simulink model "Simulation_v2"  (R2020a)
settings: Solver=VariableStepAuto  StartTime=0.0  StopTime=tmax  RelTol=1e-3
values from neighbouring files (symbols this model uses):
  BPden = [1 alpha]    [RunSimulation.m]    (also in RunTest.m)
  BPnum = [0.3 alpha]    [RunSimulation.m]    (also in RunTest.m)
  c = 250    [RunSimulation.m]    (also in RunTest.m)
  fc = 0.45    [RunTest.m]
  Ft = 360000    [RunTest.m]
  l = 18    [RunSimulation.m]    (also in RunTest.m)
  num_wagons = 10    [RunTest.m]
  p0 = 0    [RunSimulation.m]    (also in RunTest.m)
  pool = readmatrix('pool.csv')    [RunTest.m]
  Pres = 0/1000*[5.7/771 0 1.6]    [RunSimulation.m]    (also in RunTest.m)
  RBD = 5    [RunSimulation.m]    (also in RunTest.m)
  tl = .1    (= 0.1)    [RunSimulation.m]    (also in RunTest.m)
  trackgradient = 0    [RunTest.m]
  v0 = 100/3.6    (= 27.7777777778)    [RunSimulation.m]
  VBD = 3.5    [RunSimulation.m]    (also in RunTest.m)
libraries: simulink x43, commrandsrc3 x40
(part 1 of 4)
settings Model: SimulationMode=accelerator  Creator=raphael  LastModifiedBy=Westfechtel
settings SolverCC: ZeroCrossControl=DisableAll
settings DataIOCC: ReturnWorkspaceOutputs=off
settings DebuggingCC: ArithmeticOperatorsInVariantConditions=warning
settings SFSimCC: CustomCodeUndefinedFunction=UseInterfaceOnly

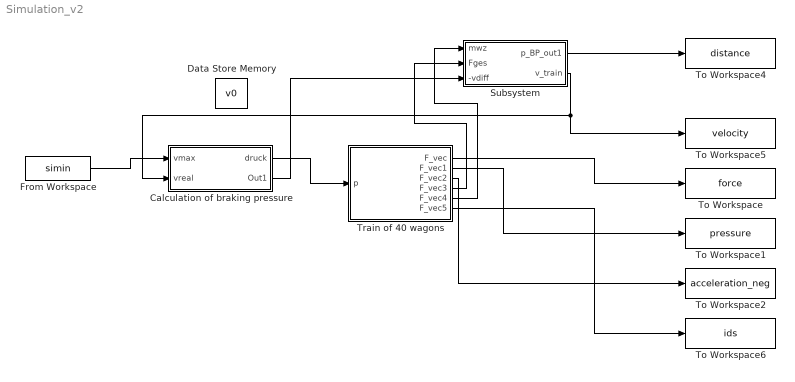
== system Simulation_v2 ==
  Calculation of braking pressure : Subsystem
  Data Store Memory : DataStoreMemory  DataStoreName=v0  ReadBeforeWriteMsg=warning  WriteAfterWriteMsg=warning  WriteAfterReadMsg=warning  ShowAdditionalParam=off
  From Workspace : FromWorkspace  VariableName=simin
  Subsystem : Subsystem
  To Workspace : ToWorkspace  VariableName=force  SaveFormat=Timeseries  SampleTime=-1
  To Workspace1 : ToWorkspace  VariableName=pressure  SaveFormat=Timeseries  SampleTime=-1
  To Workspace2 : ToWorkspace  VariableName=acceleration_neg  SaveFormat=Timeseries  SampleTime=-1
  To Workspace4 : ToWorkspace  VariableName=distance  SaveFormat=Timeseries  SampleTime=-1
  To Workspace5 : ToWorkspace  VariableName=velocity  SaveFormat=Timeseries  SampleTime=-1
  To Workspace6 : ToWorkspace  VariableName=ids  SampleTime=-1
  Train of 40 wagons : Subsystem
  wires:
  From Workspace/1 -> Calculation of braking pressure/1("vmax ")
  Calculation of braking pressure/1(druck) -> Train of 40 wagons/1(p)
  Subsystem/1(p_BP_out1) -> To Workspace4/1
  Subsystem/2(v_train) -> Calculation of braking pressure/2(vreal), To Workspace5/1
  Train of 40 wagons/1(F_vec) -> To Workspace/1
  Train of 40 wagons/2(F_vec1) -> To Workspace1/1
  Train of 40 wagons/3(F_vec2) -> To Workspace2/1
  Train of 40 wagons/4(F_vec3) -> Subsystem/2(Fges)
  Train of 40 wagons/5(F_vec4) -> Subsystem/1(mwz)
  Calculation of braking pressure/2(Out1) -> Subsystem/3("-vdiff ")
  Train of 40 wagons/6(F_vec5) -> To Workspace6/1

== system Simulation_v2/Calculation of braking pressure ==
  "vmax " : Inport
  vreal : Inport  Port=2
  1-D Lookup Table : Lookup_n-D  NumberOfTableDimensions=1  BreakpointsForDimension1=[1,2,5,10,15,20,25,30]  Table=[0.1,0.2,0.5,0.7,0.8,1,1.2,1.5]  InternalRulePriority=Speed  RndMeth=Simplest  InputSameDT=on
  Add : Sum  Inputs=+-
  Add1 : Sum
  Bias : Bias  Bias=-RBD
  Constant : Constant  Value=RBD
  Data Store Read : DataStoreRead  DataStoreName=v0
  Data Store Write : DataStoreWrite  DataStoreName=v0
  Detect Decrease : simulink/Logic and Bit Operations/Detect Decrease  vinit=0.0  OutDataTypeStr=boolean
  Divide : Product  Inputs=**
  Divide1 : Product  Inputs=**
  Gain : Gain  Gain=-1
  Logical Operator : Logic  Operator=NOT  Inputs=1  AllPortsSameDT=off  OutDataTypeStr=boolean
  Product : Product
  Relational Operator : RelationalOperator  Operator=>  OutDataTypeStr=boolean  RndMeth=Simplest
  Subtract : Sum  Inputs=+-
  To Workspace : ToWorkspace  VariableName=v0_out  SaveFormat=Timeseries  SampleTime=-1
  druck : Outport
  Out1 : Outport  Port=2
  wires:
  "vmax "/1 -> Subtract/2, Detect Decrease/1, Relational Operator/2
  Constant/1 -> Add/1
  Add/1 -> Bias/1
  Bias/1 -> druck/1
  Detect Decrease/1 -> Logical Operator/1, Divide/2
  Logical Operator/1 -> Divide1/1
  Data Store Read/1 -> Divide1/2
  Divide/1 -> Add1/1
  Divide1/1 -> Add1/2
  Add1/1 -> To Workspace/1, Data Store Write/1
  vreal/1 -> Relational Operator/1, Subtract/1, Divide/1
  Relational Operator/1 -> Product/1
  Subtract/1 -> Gain/1, 1-D Lookup Table/1
  1-D Lookup Table/1 -> Product/2
  Product/1 -> Add/2
  Gain/1 -> Out1/1

== system Simulation_v2/Subsystem ==
  mwz : Inport
  Fges : Inport  Port=2
  "-vdiff " : Inport  Port=3
  1-D Lookup Table : Lookup_n-D  NumberOfTableDimensions=1  BreakpointsForDimension1=[1,2,5,10,15,20,25,30]  Table=[0.05,0.1,0.15,0.3,0.45,0.6,0.85,1]  InternalRulePriority=Speed  RndMeth=Simplest  InputSameDT=on
  Add : Sum
  Compare To Zero : simulink/Logic and Bit Operations/Compare To Zero  relop=~=  OutDataTypeStr=boolean
  Compare To Zero1 : simulink/Logic and Bit Operations/Compare To Zero  relop===  OutDataTypeStr=boolean
  Constant : Constant  Value=Ft
  Data Store Read : DataStoreRead  DataStoreName=v0
  Dead Zone : DeadZone  LowerValue=-0.05  UpperValue=0.05  SaturateOnIntegerOverflow=on
  Divide1 : Product  Inputs=**
  Divide2 : Product  Inputs=**
  Divide3 : Product  Inputs=**
  Integrator : Integrator  InitialConditionSource=external  InitialCondition=v0
  Integrator1 : Integrator
  Mux4 : Mux  Inputs=1
  a=F/m : Product  Inputs=*/
  p_BP_out1 : Outport  VectorParamsAs1DForOutWhenUnconnected=off
  v_train : Outport  Port=2
  wires:
  Integrator1/1 -> Mux4/1
  Integrator/1 -> v_train/1, Integrator1/1  "v"
  a=F/m/1 -> Integrator/1  "a"
  Mux4/1 -> p_BP_out1/1  "distance_vec"
  mwz/1 -> a=F/m/2
  Data Store Read/1 -> Integrator/2
  Fges/1 -> Dead Zone/1
  Compare To Zero/1 -> Divide1/1
  Compare To Zero1/1 -> Divide2/2
  Divide1/1 -> Add/2
  Add/1 -> a=F/m/1
  Dead Zone/1 -> Compare To Zero1/1, Compare To Zero/1, Divide1/2
  Divide2/1 -> Add/1
  "-vdiff "/1 -> 1-D Lookup Table/1
  1-D Lookup Table/1 -> Divide3/2
  Divide3/1 -> Divide2/1
  Constant/1 -> Divide3/1

== system Simulation_v2/Train of 40 wagons ==
  p : Inport
  Add : Sum  Inputs=++++++++
  Add1 : Sum  Inputs=++++++++
  Mux{,1..3} (4 alike) : Mux  Inputs=8
  Subsystem1 : Subsystem
  Subsystem2 : Subsystem
  Subsystem3 : Subsystem
  Subsystem4 : Subsystem
  Subsystem5 : Subsystem
  Subsystem6 : Subsystem
  Subsystem7 : Subsystem
  Subsystem8 : Subsystem
  Terminator : Terminator
  F_vec : Outport  VectorParamsAs1DForOutWhenUnconnected=off
  F_vec1 : Outport  Port=2  VectorParamsAs1DForOutWhenUnconnected=off
  F_vec2 : Outport  Port=3  VectorParamsAs1DForOutWhenUnconnected=off
  F_vec3 : Outport  Port=4  VectorParamsAs1DForOutWhenUnconnected=off
  F_vec4 : Outport  Port=5  VectorParamsAs1DForOutWhenUnconnected=off
  F_vec5 : Outport  Port=6  VectorParamsAs1DForOutWhenUnconnected=off
  wires:
  p/1 -> Subsystem1/1(In1)
  Mux/1 -> F_vec/1  "F_vec"
  Mux1/1 -> F_vec1/1  "BP_vec"
  Mux2/1 -> F_vec2/1  "ares_vec"
  Add/1 -> F_vec3/1  "Fges"
  Add1/1 -> F_vec4/1  "mwz"
  Subsystem1/1(F_vec) -> Mux/1
  Subsystem2/1(F_vec) -> Mux/2
  Subsystem3/1(F_vec) -> Mux/3
  Subsystem4/1(F_vec) -> Mux/4
  Subsystem5/1(F_vec) -> Mux/5
  Subsystem6/1(F_vec) -> Mux/6
  Subsystem8/1(F_vec) -> Mux/7
  Subsystem7/1(F_vec) -> Mux/8
  Subsystem1/2(BP_vec) -> Mux1/1
  Subsystem2/2(BP_vec) -> Mux1/2
  Subsystem3/2(BP_vec) -> Mux1/3
  Subsystem4/2(BP_vec) -> Mux1/4
  Subsystem5/2(BP_vec) -> Mux1/5
  Subsystem6/2(BP_vec) -> Mux1/6
  Subsystem8/2(BP_vec) -> Mux1/7
  Subsystem7/2(BP_vec) -> Mux1/8
  Subsystem1/3(ares_vec) -> Mux2/1
  Subsystem2/3(ares_vec) -> Mux2/2
  Subsystem3/3(ares_vec) -> Mux2/3
  Subsystem4/3(ares_vec) -> Mux2/4
  Subsystem5/3(ares_vec) -> Mux2/5
  Subsystem6/3(ares_vec) -> Mux2/6
  Subsystem8/3(ares_vec) -> Mux2/7
  Subsystem7/3(ares_vec) -> Mux2/8
  Subsystem1/4(p_BP_out) -> Subsystem2/1(In1)
  Subsystem2/4(p_BP_out) -> Subsystem3/1(In1)
  Subsystem3/4(p_BP_out) -> Subsystem4/1(In1)
  Subsystem4/4(p_BP_out) -> Subsystem5/1(In1)
  Subsystem5/4(p_BP_out) -> Subsystem6/1(In1)
  Subsystem6/4(p_BP_out) -> Subsystem8/1(In1)
  Subsystem8/4(p_BP_out) -> Subsystem7/1(In1)
  Subsystem7/4(p_BP_out) -> Terminator/1
  Subsystem1/5(BP_vec1) -> Add/1
  Subsystem2/5(BP_vec1) -> Add/2
  Subsystem3/5(BP_vec1) -> Add/3
  Subsystem4/5(BP_vec1) -> Add/4
  Subsystem5/5(BP_vec1) -> Add/5
  Subsystem6/5(BP_vec1) -> Add/6
  Subsystem8/5(BP_vec1) -> Add/7
  Subsystem7/5(BP_vec1) -> Add/8
  Subsystem1/6(BP_vec2) -> Add1/1
  Subsystem2/6(BP_vec2) -> Add1/2
  Subsystem3/6(BP_vec2) -> Add1/3
  Subsystem4/6(BP_vec2) -> Add1/4
  Subsystem5/6(BP_vec2) -> Add1/5
  Subsystem6/6(BP_vec2) -> Add1/6
  Subsystem8/6(BP_vec2) -> Add1/7
  Subsystem7/6(BP_vec2) -> Add1/8
  Mux3/1 -> F_vec5/1  "id_vec"
  Subsystem1/7(ares_vec1) -> Mux3/1
  Subsystem2/7(ares_vec1) -> Mux3/2
  Subsystem3/7(ares_vec1) -> Mux3/3
  Subsystem4/7(ares_vec1) -> Mux3/4
  Subsystem5/7(ares_vec1) -> Mux3/5
  Subsystem6/7(ares_vec1) -> Mux3/6
  Subsystem8/7(ares_vec1) -> Mux3/7
  Subsystem7/7(ares_vec1) -> Mux3/8

== system Simulation_v2/Train of 40 wagons/Subsystem1 ==
  In1 : Inport
  Add : Sum  Inputs=+++++
  Add1 : Sum  Inputs=+++++
  Mux{,1..3} (4 alike) : Mux  Inputs=5
  Wagon model1 : Subsystem
  Wagon model2 : Subsystem
  Wagon model3 : Subsystem
  Wagon model4 : Subsystem
  Wagon model5 : Subsystem
  F_vec : Outport  VectorParamsAs1DForOutWhenUnconnected=off
  BP_vec : Outport  Port=2  VectorParamsAs1DForOutWhenUnconnected=off
  ares_vec : Outport  Port=3  VectorParamsAs1DForOutWhenUnconnected=off
  p_BP_out : Outport  Port=4  VectorParamsAs1DForOutWhenUnconnected=off
  BP_vec1 : Outport  Port=5  VectorParamsAs1DForOutWhenUnconnected=off
  BP_vec2 : Outport  Port=6  VectorParamsAs1DForOutWhenUnconnected=off
  ares_vec1 : Outport  Port=7  VectorParamsAs1DForOutWhenUnconnected=off
  wires:
  In1/1 -> Wagon model5/1(p)
  Mux1/1 -> BP_vec/1  "BP_vec"
  Mux/1 -> F_vec/1  "F_vec"
  Mux3/1 -> ares_vec/1  "ares_vec"
  Add1/1 -> BP_vec2/1  "msum"
  Add/1 -> BP_vec1/1  "Fsum"
  Wagon model5/2(p_BP_out) -> Wagon model3/1(p), Mux1/1  "p_BP_out"
  Wagon model3/2(p_BP_out) -> Wagon model2/1(p), Mux1/2  "p_BP_out"
  Wagon model2/2(p_BP_out) -> Wagon model1/1(p), Mux1/3  "p_BP_out"
  Wagon model1/2(p_BP_out) -> Wagon model4/1(p), Mux1/4  "p_BP_out"
  Wagon model4/2(p_BP_out) -> Mux1/5, p_BP_out/1  "p_BP_out"
  Wagon model5/1(Fres) -> Add/1, Mux/1
  Wagon model3/1(Fres) -> Add/2, Mux/2
  Wagon model2/1(Fres) -> Mux/3, Add/3
  Wagon model1/1(Fres) -> Mux/4, Add/4
  Wagon model4/1(Fres) -> Mux/5, Add/5
  Wagon model5/3(ares) -> Mux3/1
  Wagon model3/3(ares) -> Mux3/2
  Wagon model2/3(ares) -> Mux3/3
  Wagon model1/3(ares) -> Mux3/4
  Wagon model4/3(ares) -> Mux3/5
  Wagon model5/4(m) -> Add1/1
  Wagon model3/4(m) -> Add1/2
  Wagon model2/4(m) -> Add1/3
  Wagon model1/4(m) -> Add1/4
  Wagon model4/4(m) -> Add1/5
  Mux2/1 -> ares_vec1/1  "id_vec"
  Wagon model5/5("id ") -> Mux2/1
  Wagon model3/5("id ") -> Mux2/2
  Wagon model2/5("id ") -> Mux2/3
  Wagon model1/5("id ") -> Mux2/4
  Wagon model4/5("id ") -> Mux2/5

== system Simulation_v2/Train of 40 wagons/Subsystem2 ==
  In1 : Inport
  Add : Sum  Inputs=+++++
  Add1 : Sum  Inputs=+++++
  Mux{,1..3} (4 alike) : Mux  Inputs=5
  Wagon model1 : Subsystem
  Wagon model2 : Subsystem
  Wagon model3 : Subsystem
  Wagon model4 : Subsystem
  Wagon model5 : Subsystem
  F_vec : Outport  VectorParamsAs1DForOutWhenUnconnected=off
  BP_vec : Outport  Port=2  VectorParamsAs1DForOutWhenUnconnected=off
  ares_vec : Outport  Port=3  VectorParamsAs1DForOutWhenUnconnected=off
  p_BP_out : Outport  Port=4  VectorParamsAs1DForOutWhenUnconnected=off
  BP_vec1 : Outport  Port=5  VectorParamsAs1DForOutWhenUnconnected=off
  BP_vec2 : Outport  Port=6  VectorParamsAs1DForOutWhenUnconnected=off
  ares_vec1 : Outport  Port=7  VectorParamsAs1DForOutWhenUnconnected=off
  wires:
  In1/1 -> Wagon model5/1(p)
  Mux1/1 -> BP_vec/1  "BP_vec"
  Mux/1 -> F_vec/1  "F_vec"
  Mux3/1 -> ares_vec/1  "ares_vec"
  Add1/1 -> BP_vec2/1  "msum"
  Add/1 -> BP_vec1/1  "Fsum"
  Wagon model5/2(p_BP_out) -> Wagon model3/1(p), Mux1/1  "p_BP_out"
  Wagon model3/2(p_BP_out) -> Wagon model2/1(p), Mux1/2  "p_BP_out"
  Wagon model2/2(p_BP_out) -> Wagon model1/1(p), Mux1/3  "p_BP_out"
  Wagon model1/2(p_BP_out) -> Wagon model4/1(p), Mux1/4  "p_BP_out"
  Wagon model4/2(p_BP_out) -> Mux1/5, p_BP_out/1  "p_BP_out"
  Wagon model5/1(Fres) -> Add/1, Mux/1
  Wagon model3/1(Fres) -> Add/2, Mux/2
  Wagon model2/1(Fres) -> Mux/3, Add/3
  Wagon model1/1(Fres) -> Mux/4, Add/4
  Wagon model4/1(Fres) -> Mux/5, Add/5
  Wagon model5/3(ares) -> Mux3/1
  Wagon model3/3(ares) -> Mux3/2
  Wagon model2/3(ares) -> Mux3/3
  Wagon model1/3(ares) -> Mux3/4
  Wagon model4/3(ares) -> Mux3/5
  Wagon model5/4(m) -> Add1/1
  Wagon model3/4(m) -> Add1/2
  Wagon model2/4(m) -> Add1/3
  Wagon model1/4(m) -> Add1/4
  Wagon model4/4(m) -> Add1/5
  Mux2/1 -> ares_vec1/1  "id_vec"
  Wagon model5/5("id ") -> Mux2/1
  Wagon model3/5("id ") -> Mux2/2
  Wagon model2/5("id ") -> Mux2/3
  Wagon model1/5("id ") -> Mux2/4
  Wagon model4/5("id ") -> Mux2/5

== system Simulation_v2/Train of 40 wagons/Subsystem3 ==
  In1 : Inport
  Add : Sum  Inputs=+++++
  Add1 : Sum  Inputs=+++++
  Mux{,1..3} (4 alike) : Mux  Inputs=5
  Wagon model1 : Subsystem
  Wagon model2 : Subsystem
  Wagon model3 : Subsystem
  Wagon model4 : Subsystem
  Wagon model5 : Subsystem
  F_vec : Outport  VectorParamsAs1DForOutWhenUnconnected=off
  BP_vec : Outport  Port=2  VectorParamsAs1DForOutWhenUnconnected=off
  ares_vec : Outport  Port=3  VectorParamsAs1DForOutWhenUnconnected=off
  p_BP_out : Outport  Port=4  VectorParamsAs1DForOutWhenUnconnected=off
  BP_vec1 : Outport  Port=5  VectorParamsAs1DForOutWhenUnconnected=off
  BP_vec2 : Outport  Port=6  VectorParamsAs1DForOutWhenUnconnected=off
  ares_vec1 : Outport  Port=7  VectorParamsAs1DForOutWhenUnconnected=off
  wires:
  In1/1 -> Wagon model5/1(p)
  Mux1/1 -> BP_vec/1  "BP_vec"
  Mux/1 -> F_vec/1  "F_vec"
  Mux3/1 -> ares_vec/1  "ares_vec"
  Add1/1 -> BP_vec2/1  "msum"
  Add/1 -> BP_vec1/1  "Fsum"
  Wagon model5/2(p_BP_out) -> Wagon model3/1(p), Mux1/1  "p_BP_out"
  Wagon model3/2(p_BP_out) -> Wagon model2/1(p), Mux1/2  "p_BP_out"
  Wagon model2/2(p_BP_out) -> Wagon model1/1(p), Mux1/3  "p_BP_out"
  Wagon model1/2(p_BP_out) -> Wagon model4/1(p), Mux1/4  "p_BP_out"
  Wagon model4/2(p_BP_out) -> Mux1/5, p_BP_out/1  "p_BP_out"
  Wagon model5/1(Fres) -> Add/1, Mux/1
  Wagon model3/1(Fres) -> Add/2, Mux/2
  Wagon model2/1(Fres) -> Mux/3, Add/3
  Wagon model1/1(Fres) -> Mux/4, Add/4
  Wagon model4/1(Fres) -> Mux/5, Add/5
  Wagon model5/3(ares) -> Mux3/1
  Wagon model3/3(ares) -> Mux3/2
  Wagon model2/3(ares) -> Mux3/3
  Wagon model1/3(ares) -> Mux3/4
  Wagon model4/3(ares) -> Mux3/5
  Wagon model5/4(m) -> Add1/1
  Wagon model3/4(m) -> Add1/2
  Wagon model2/4(m) -> Add1/3
  Wagon model1/4(m) -> Add1/4
  Wagon model4/4(m) -> Add1/5
  Mux2/1 -> ares_vec1/1  "id_vec"
  Wagon model5/5("id ") -> Mux2/1
  Wagon model3/5("id ") -> Mux2/2
  Wagon model2/5("id ") -> Mux2/3
  Wagon model1/5("id ") -> Mux2/4
  Wagon model4/5("id ") -> Mux2/5

== system Simulation_v2/Train of 40 wagons/Subsystem4 ==
  In1 : Inport
  Add : Sum  Inputs=+++++
  Add1 : Sum  Inputs=+++++
  Mux{,1..3} (4 alike) : Mux  Inputs=5
  Wagon model1 : Subsystem
  Wagon model2 : Subsystem
  Wagon model3 : Subsystem
  Wagon model4 : Subsystem
  Wagon model5 : Subsystem
  F_vec : Outport  VectorParamsAs1DForOutWhenUnconnected=off
  BP_vec : Outport  Port=2  VectorParamsAs1DForOutWhenUnconnected=off
  ares_vec : Outport  Port=3  VectorParamsAs1DForOutWhenUnconnected=off
  p_BP_out : Outport  Port=4  VectorParamsAs1DForOutWhenUnconnected=off
  BP_vec1 : Outport  Port=5  VectorParamsAs1DForOutWhenUnconnected=off
  BP_vec2 : Outport  Port=6  VectorParamsAs1DForOutWhenUnconnected=off
  ares_vec1 : Outport  Port=7  VectorParamsAs1DForOutWhenUnconnected=off
  wires:
  In1/1 -> Wagon model5/1(p)
  Mux1/1 -> BP_vec/1  "BP_vec"
  Mux/1 -> F_vec/1  "F_vec"
  Mux3/1 -> ares_vec/1  "ares_vec"
  Add1/1 -> BP_vec2/1  "msum"
  Add/1 -> BP_vec1/1  "Fsum"
  Wagon model5/2(p_BP_out) -> Wagon model3/1(p), Mux1/1  "p_BP_out"
  Wagon model3/2(p_BP_out) -> Wagon model2/1(p), Mux1/2  "p_BP_out"
  Wagon model2/2(p_BP_out) -> Wagon model1/1(p), Mux1/3  "p_BP_out"
  Wagon model1/2(p_BP_out) -> Wagon model4/1(p), Mux1/4  "p_BP_out"
  Wagon model4/2(p_BP_out) -> Mux1/5, p_BP_out/1  "p_BP_out"
  Wagon model5/1(Fres) -> Add/1, Mux/1
  Wagon model3/1(Fres) -> Add/2, Mux/2
  Wagon model2/1(Fres) -> Mux/3, Add/3
  Wagon model1/1(Fres) -> Mux/4, Add/4
  Wagon model4/1(Fres) -> Mux/5, Add/5
  Wagon model5/3(ares) -> Mux3/1
  Wagon model3/3(ares) -> Mux3/2
  Wagon model2/3(ares) -> Mux3/3
  Wagon model1/3(ares) -> Mux3/4
  Wagon model4/3(ares) -> Mux3/5
  Wagon model5/4(m) -> Add1/1
  Wagon model3/4(m) -> Add1/2
  Wagon model2/4(m) -> Add1/3
  Wagon model1/4(m) -> Add1/4
  Wagon model4/4(m) -> Add1/5
  Mux2/1 -> ares_vec1/1  "id_vec"
  Wagon model5/5("id ") -> Mux2/1
  Wagon model3/5("id ") -> Mux2/2
  Wagon model2/5("id ") -> Mux2/3
  Wagon model1/5("id ") -> Mux2/4
  Wagon model4/5("id ") -> Mux2/5

== system Simulation_v2/Train of 40 wagons/Subsystem5 ==
  In1 : Inport
  Add : Sum  Inputs=+++++
  Add1 : Sum  Inputs=+++++
  Mux{,1..3} (4 alike) : Mux  Inputs=5
  Wagon model1 : Subsystem
  Wagon model2 : Subsystem
  Wagon model3 : Subsystem
  Wagon model4 : Subsystem
  Wagon model5 : Subsystem
  F_vec : Outport  VectorParamsAs1DForOutWhenUnconnected=off
  BP_vec : Outport  Port=2  VectorParamsAs1DForOutWhenUnconnected=off
  ares_vec : Outport  Port=3  VectorParamsAs1DForOutWhenUnconnected=off
  p_BP_out : Outport  Port=4  VectorParamsAs1DForOutWhenUnconnected=off
  BP_vec1 : Outport  Port=5  VectorParamsAs1DForOutWhenUnconnected=off
  BP_vec2 : Outport  Port=6  VectorParamsAs1DForOutWhenUnconnected=off
  ares_vec1 : Outport  Port=7  VectorParamsAs1DForOutWhenUnconnected=off
  wires:
  In1/1 -> Wagon model5/1(p)
  Mux1/1 -> BP_vec/1  "BP_vec"
  Mux/1 -> F_vec/1  "F_vec"
  Mux3/1 -> ares_vec/1  "ares_vec"
  Add1/1 -> BP_vec2/1  "msum"
  Add/1 -> BP_vec1/1  "Fsum"
  Wagon model5/2(p_BP_out) -> Wagon model3/1(p), Mux1/1  "p_BP_out"
  Wagon model3/2(p_BP_out) -> Wagon model2/1(p), Mux1/2  "p_BP_out"
  Wagon model2/2(p_BP_out) -> Wagon model1/1(p), Mux1/3  "p_BP_out"
  Wagon model1/2(p_BP_out) -> Wagon model4/1(p), Mux1/4  "p_BP_out"
  Wagon model4/2(p_BP_out) -> Mux1/5, p_BP_out/1  "p_BP_out"
  Wagon model5/1(Fres) -> Add/1, Mux/1
  Wagon model3/1(Fres) -> Add/2, Mux/2
  Wagon model2/1(Fres) -> Mux/3, Add/3
  Wagon model1/1(Fres) -> Mux/4, Add/4
  Wagon model4/1(Fres) -> Mux/5, Add/5
  Wagon model5/3(ares) -> Mux3/1
  Wagon model3/3(ares) -> Mux3/2
  Wagon model2/3(ares) -> Mux3/3
  Wagon model1/3(ares) -> Mux3/4
  Wagon model4/3(ares) -> Mux3/5
  Wagon model5/4(m) -> Add1/1
  Wagon model3/4(m) -> Add1/2
  Wagon model2/4(m) -> Add1/3
  Wagon model1/4(m) -> Add1/4
  Wagon model4/4(m) -> Add1/5
  Mux2/1 -> ares_vec1/1  "id_vec"
  Wagon model5/5("id ") -> Mux2/1
  Wagon model3/5("id ") -> Mux2/2
  Wagon model2/5("id ") -> Mux2/3
  Wagon model1/5("id ") -> Mux2/4
  Wagon model4/5("id ") -> Mux2/5

== system Simulation_v2/Train of 40 wagons/Subsystem6 ==
  In1 : Inport
  Add : Sum  Inputs=+++++
  Add1 : Sum  Inputs=+++++
  Mux{,1..3} (4 alike) : Mux  Inputs=5
  Wagon model1 : Subsystem
  Wagon model2 : Subsystem
  Wagon model3 : Subsystem
  Wagon model4 : Subsystem
  Wagon model5 : Subsystem
  F_vec : Outport  VectorParamsAs1DForOutWhenUnconnected=off
  BP_vec : Outport  Port=2  VectorParamsAs1DForOutWhenUnconnected=off
  ares_vec : Outport  Port=3  VectorParamsAs1DForOutWhenUnconnected=off
  p_BP_out : Outport  Port=4  VectorParamsAs1DForOutWhenUnconnected=off
  BP_vec1 : Outport  Port=5  VectorParamsAs1DForOutWhenUnconnected=off
  BP_vec2 : Outport  Port=6  VectorParamsAs1DForOutWhenUnconnected=off
  ares_vec1 : Outport  Port=7  VectorParamsAs1DForOutWhenUnconnected=off
  wires:
  In1/1 -> Wagon model5/1(p)
  Mux1/1 -> BP_vec/1  "BP_vec"
  Mux/1 -> F_vec/1  "F_vec"
  Mux3/1 -> ares_vec/1  "ares_vec"
  Add1/1 -> BP_vec2/1  "msum"
  Add/1 -> BP_vec1/1  "Fsum"
  Wagon model5/2(p_BP_out) -> Wagon model3/1(p), Mux1/1  "p_BP_out"
  Wagon model3/2(p_BP_out) -> Wagon model2/1(p), Mux1/2  "p_BP_out"
  Wagon model2/2(p_BP_out) -> Wagon model1/1(p), Mux1/3  "p_BP_out"
  Wagon model1/2(p_BP_out) -> Wagon model4/1(p), Mux1/4  "p_BP_out"
  Wagon model4/2(p_BP_out) -> Mux1/5, p_BP_out/1  "p_BP_out"
  Wagon model5/1(Fres) -> Add/1, Mux/1
  Wagon model3/1(Fres) -> Add/2, Mux/2
  Wagon model2/1(Fres) -> Mux/3, Add/3
  Wagon model1/1(Fres) -> Mux/4, Add/4
  Wagon model4/1(Fres) -> Mux/5, Add/5
  Wagon model5/3(ares) -> Mux3/1
  Wagon model3/3(ares) -> Mux3/2
  Wagon model2/3(ares) -> Mux3/3
  Wagon model1/3(ares) -> Mux3/4
  Wagon model4/3(ares) -> Mux3/5
  Wagon model5/4(m) -> Add1/1
  Wagon model3/4(m) -> Add1/2
  Wagon model2/4(m) -> Add1/3
  Wagon model1/4(m) -> Add1/4
  Wagon model4/4(m) -> Add1/5
  Mux2/1 -> ares_vec1/1  "id_vec"
  Wagon model5/5("id ") -> Mux2/1
  Wagon model3/5("id ") -> Mux2/2
  Wagon model2/5("id ") -> Mux2/3
  Wagon model1/5("id ") -> Mux2/4
  Wagon model4/5("id ") -> Mux2/5

== system Simulation_v2/Train of 40 wagons/Subsystem7 ==
  In1 : Inport
  Add : Sum  Inputs=+++++
  Add1 : Sum  Inputs=+++++
  Mux{,1..3} (4 alike) : Mux  Inputs=5
  Wagon model1 : Subsystem
  Wagon model2 : Subsystem
  Wagon model3 : Subsystem
  Wagon model4 : Subsystem
  Wagon model5 : Subsystem
  F_vec : Outport  VectorParamsAs1DForOutWhenUnconnected=off
  BP_vec : Outport  Port=2  VectorParamsAs1DForOutWhenUnconnected=off
  ares_vec : Outport  Port=3  VectorParamsAs1DForOutWhenUnconnected=off
  p_BP_out : Outport  Port=4  VectorParamsAs1DForOutWhenUnconnected=off
  BP_vec1 : Outport  Port=5  VectorParamsAs1DForOutWhenUnconnected=off
  BP_vec2 : Outport  Port=6  VectorParamsAs1DForOutWhenUnconnected=off
  ares_vec1 : Outport  Port=7  VectorParamsAs1DForOutWhenUnconnected=off
  wires:
  In1/1 -> Wagon model5/1(p)
  Mux1/1 -> BP_vec/1  "BP_vec"
  Mux/1 -> F_vec/1  "F_vec"
  Mux3/1 -> ares_vec/1  "ares_vec"
  Add1/1 -> BP_vec2/1  "msum"
  Add/1 -> BP_vec1/1  "Fsum"
  Wagon model5/2(p_BP_out) -> Wagon model3/1(p), Mux1/1  "p_BP_out"
  Wagon model3/2(p_BP_out) -> Wagon model2/1(p), Mux1/2  "p_BP_out"
  Wagon model2/2(p_BP_out) -> Wagon model1/1(p), Mux1/3  "p_BP_out"
  Wagon model1/2(p_BP_out) -> Wagon model4/1(p), Mux1/4  "p_BP_out"
  Wagon model4/2(p_BP_out) -> Mux1/5, p_BP_out/1  "p_BP_out"
  Wagon model5/1(Fres) -> Add/1, Mux/1
  Wagon model3/1(Fres) -> Add/2, Mux/2
  Wagon model2/1(Fres) -> Mux/3, Add/3
  Wagon model1/1(Fres) -> Mux/4, Add/4
  Wagon model4/1(Fres) -> Mux/5, Add/5
  Wagon model5/3(ares) -> Mux3/1
  Wagon model3/3(ares) -> Mux3/2
  Wagon model2/3(ares) -> Mux3/3
  Wagon model1/3(ares) -> Mux3/4
  Wagon model4/3(ares) -> Mux3/5
  Wagon model5/4(m) -> Add1/1
  Wagon model3/4(m) -> Add1/2
  Wagon model2/4(m) -> Add1/3
  Wagon model1/4(m) -> Add1/4
  Wagon model4/4(m) -> Add1/5
  Mux2/1 -> ares_vec1/1  "id_vec"
  Wagon model5/5("id ") -> Mux2/1
  Wagon model3/5("id ") -> Mux2/2
  Wagon model2/5("id ") -> Mux2/3
  Wagon model1/5("id ") -> Mux2/4
  Wagon model4/5("id ") -> Mux2/5

== system Simulation_v2/Train of 40 wagons/Subsystem8 ==
  In1 : Inport
  Add : Sum  Inputs=+++++
  Add1 : Sum  Inputs=+++++
  Mux{,1..3} (4 alike) : Mux  Inputs=5
  Wagon model1 : Subsystem
  Wagon model2 : Subsystem
  Wagon model3 : Subsystem
  Wagon model4 : Subsystem
  Wagon model5 : Subsystem
  F_vec : Outport  VectorParamsAs1DForOutWhenUnconnected=off
  BP_vec : Outport  Port=2  VectorParamsAs1DForOutWhenUnconnected=off
  ares_vec : Outport  Port=3  VectorParamsAs1DForOutWhenUnconnected=off
  p_BP_out : Outport  Port=4  VectorParamsAs1DForOutWhenUnconnected=off
  BP_vec1 : Outport  Port=5  VectorParamsAs1DForOutWhenUnconnected=off
  BP_vec2 : Outport  Port=6  VectorParamsAs1DForOutWhenUnconnected=off
  ares_vec1 : Outport  Port=7  VectorParamsAs1DForOutWhenUnconnected=off
  wires:
  In1/1 -> Wagon model5/1(p)
  Mux1/1 -> BP_vec/1  "BP_vec"
  Mux/1 -> F_vec/1  "F_vec"
  Mux3/1 -> ares_vec/1  "ares_vec"
  Add1/1 -> BP_vec2/1  "msum"
  Add/1 -> BP_vec1/1  "Fsum"
  Wagon model5/2(p_BP_out) -> Wagon model3/1(p), Mux1/1  "p_BP_out"
  Wagon model3/2(p_BP_out) -> Wagon model2/1(p), Mux1/2  "p_BP_out"
  Wagon model2/2(p_BP_out) -> Wagon model1/1(p), Mux1/3  "p_BP_out"
  Wagon model1/2(p_BP_out) -> Wagon model4/1(p), Mux1/4  "p_BP_out"
  Wagon model4/2(p_BP_out) -> Mux1/5, p_BP_out/1  "p_BP_out"
  Wagon model5/1(Fres) -> Add/1, Mux/1
  Wagon model3/1(Fres) -> Add/2, Mux/2
  Wagon model2/1(Fres) -> Mux/3, Add/3
  Wagon model1/1(Fres) -> Mux/4, Add/4
  Wagon model4/1(Fres) -> Mux/5, Add/5
  Wagon model5/3(ares) -> Mux3/1
  Wagon model3/3(ares) -> Mux3/2
  Wagon model2/3(ares) -> Mux3/3
  Wagon model1/3(ares) -> Mux3/4
  Wagon model4/3(ares) -> Mux3/5
  Wagon model5/4(m) -> Add1/1
  Wagon model3/4(m) -> Add1/2
  Wagon model2/4(m) -> Add1/3
  Wagon model1/4(m) -> Add1/4
  Wagon model4/4(m) -> Add1/5
  Mux2/1 -> ares_vec1/1  "id_vec"
  Wagon model5/5("id ") -> Mux2/1
  Wagon model3/5("id ") -> Mux2/2
  Wagon model2/5("id ") -> Mux2/3
  Wagon model1/5("id ") -> Mux2/4
  Wagon model4/5("id ") -> Mux2/5

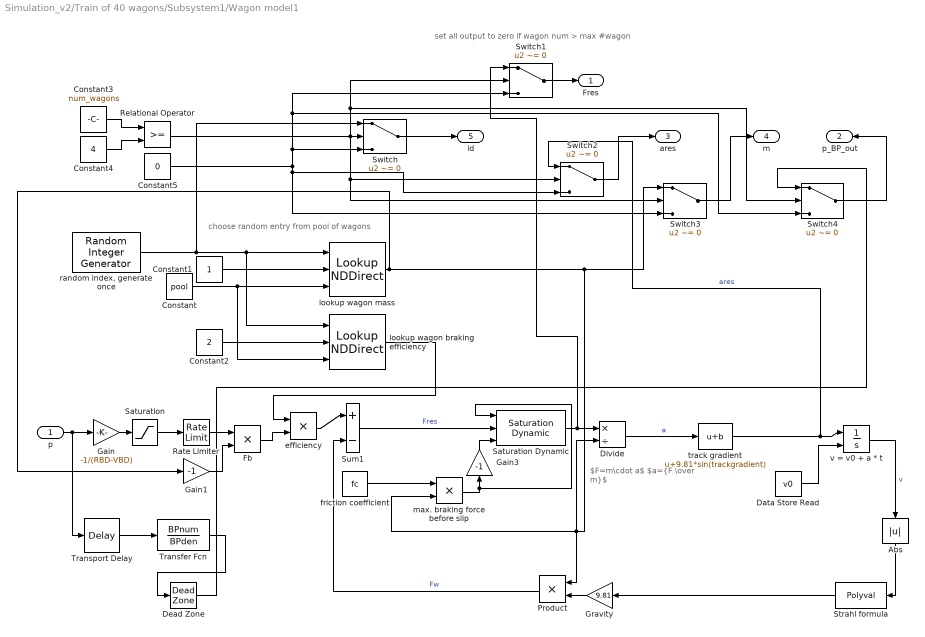
== system Simulation_v2/Train of 40 wagons/Subsystem1/Wagon model1 ==
  note: set all output to zero if wagon num > max #wagon
  note: choose random entry from pool of wagons
  note: $F=m\cdot a$ $a={F \over m}$
  p : Inport
  Abs : Abs
  Constant : Constant  Value=pool
  Constant1 : Constant
  Constant2 : Constant  Value=2
  Constant3 : Constant  Value=num_wagons
  Constant4 : Constant  Value=4
  Constant5 : Constant  Value=0  OutDataTypeStr=uint32
  Data Store Read : DataStoreRead  DataStoreName=v0
  Dead Zone : DeadZone  LowerValue=-0.005  UpperValue=0.005  SaturateOnIntegerOverflow=on
  Divide : Product  Inputs=*/
  Fb : Product  Inputs=**
  Gain : Gain  Gain=-1/(RBD-VBD)
  Gain1 : Gain  Gain=-1
  Gain3 : Gain  Gain=-1
  Gravity : Gain  Gain=9.81
  Product : Product
  Rate Limiter : RateLimiter  RisingSlewLimit=1/tf  FallingSlewLimit=-1/tl  SampleTimeMode=inherited
  Relational Operator : RelationalOperator  OutDataTypeStr=boolean  RndMeth=Simplest
  Saturation : Saturate  UpperLimit=1  LowerLimit=0
  Saturation Dynamic : simulink/Discontinuities/Saturation Dynamic  OutMin=[]  OutMax=[]  OutDataTypeStr=Inherit: Same as second input  OutDataType=fixdt(1, 16)  OutScaling=2^-10  DoSatur=off
  Strahl formula : Polyval  Coefs=Pres
  Sum1 : Sum  Inputs=|+-
  Switch{,1..4} (5 alike) : Switch  Criteria=u2 ~= 0
  Transfer Fcn : TransferFcn  Numerator=BPnum  Denominator=BPden
  Transport Delay : TransportDelay  DelayTime=l/c  InitialOutput=p0
  efficiency : Product  Inputs=**
  friction coefficient : Constant  Value=fc
  lookup wagon braking efficiency : LookupNDDirect  TableIsInput=on
  lookup wagon mass : LookupNDDirect  TableIsInput=on
  max. braking force before slip : Product  Inputs=**
  "random index, generate once " : commrandsrc3/Random Integer Generator  SetSize=500  SeedSource=Auto  Seed=0  SampleTime=999999  SamplesPerFrame=1  OutputDataType=uint32  SimulateUsing=Interpreted execution
  track gradient : Bias  Bias=9.81*sin(trackgradient)
  v = v0 + a * t : Integrator  InitialConditionSource=external  InitialCondition=v0
  Fres : Outport  VectorParamsAs1DForOutWhenUnconnected=off
  p_BP_out : Outport  Port=2  VectorParamsAs1DForOutWhenUnconnected=off
  ares : Outport  Port=3
  m : Outport  Port=4
  "id " : Outport  Port=5
  wires:
  Strahl formula/1 -> Gravity/1
  Abs/1 -> Strahl formula/1
  Gravity/1 -> Product/2
  Product/1 -> Sum1/2  "Fw"
  v = v0 + a * t/1 -> Abs/1  "v"
  lookup wagon mass/1 -> Gain1/1, Switch3/1, max. braking force before slip/2, Divide/2, Product/1
  Divide/1 -> track gradient/1  "a"
  Gain/1 -> Saturation/1
  Fb/1 -> efficiency/2
  Saturation/1 -> Rate Limiter/1
  Rate Limiter/1 -> Fb/1
  Transfer Fcn/1 -> Dead Zone/1
  Transport Delay/1 -> Transfer Fcn/1
  efficiency/1 -> Sum1/1
  track gradient/1 -> Switch2/1, v = v0 + a * t/1  "ares"
  p/1 -> Gain/1, Transport Delay/1
  friction coefficient/1 -> max. braking force before slip/1
  Sum1/1 -> Saturation Dynamic/2  "Fres"
  Saturation Dynamic/1 -> Switch1/1, Divide/1
  max. braking force before slip/1 -> Saturation Dynamic/1, Gain3/1
  Gain3/1 -> Saturation Dynamic/3
  Data Store Read/1 -> v = v0 + a * t/2
  Dead Zone/1 -> Switch4/1
  Constant/1 -> lookup wagon braking efficiency/3, lookup wagon mass/3
  "random index, generate once "/1 -> Switch/1, lookup wagon mass/1, lookup wagon braking efficiency/1
  Constant1/1 -> lookup wagon mass/2
  Constant2/1 -> lookup wagon braking efficiency/2
  lookup wagon braking efficiency/1 -> efficiency/1
  Gain1/1 -> Fb/2
  Constant3/1 -> Relational Operator/1
  Constant4/1 -> Relational Operator/2
  Relational Operator/1 -> Switch1/2, Switch4/2, Switch2/2, Switch3/2, Switch/2
  Switch/1 -> "id "/1
  Constant5/1 -> Switch4/3, Switch1/3, Switch/3, Switch2/3, Switch3/3
  Switch1/1 -> Fres/1
  Switch2/1 -> ares/1
  Switch3/1 -> m/1
  Switch4/1 -> p_BP_out/1

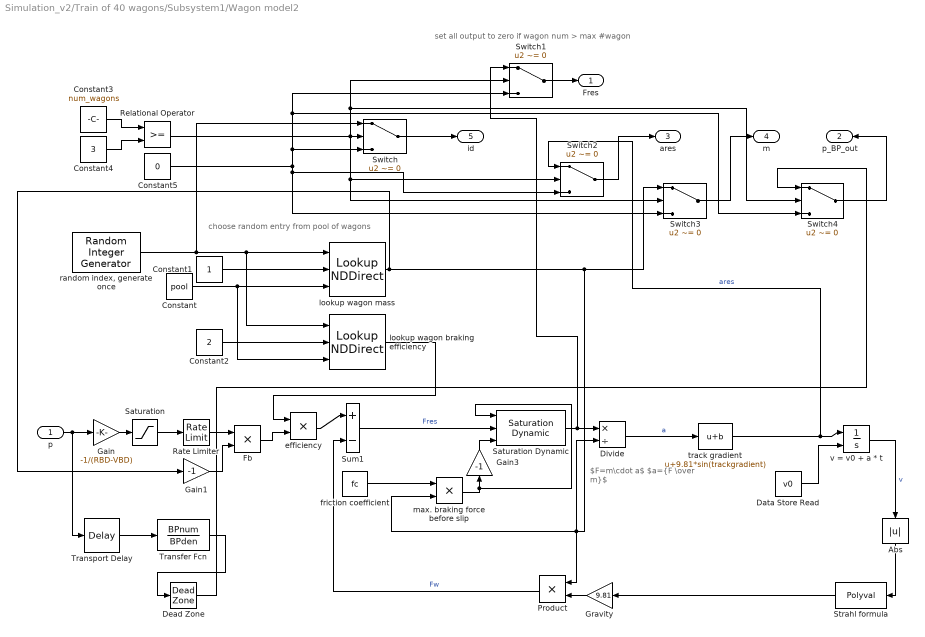
== system Simulation_v2/Train of 40 wagons/Subsystem1/Wagon model2 ==
  note: set all output to zero if wagon num > max #wagon
  note: choose random entry from pool of wagons
  note: $F=m\cdot a$ $a={F \over m}$
  p : Inport
  Abs : Abs
  Constant : Constant  Value=pool
  Constant1 : Constant
  Constant2 : Constant  Value=2
  Constant3 : Constant  Value=num_wagons
  Constant4 : Constant  Value=3
  Constant5 : Constant  Value=0  OutDataTypeStr=uint32
  Data Store Read : DataStoreRead  DataStoreName=v0
  Dead Zone : DeadZone  LowerValue=-0.005  UpperValue=0.005  SaturateOnIntegerOverflow=on
  Divide : Product  Inputs=*/
  Fb : Product  Inputs=**
  Gain : Gain  Gain=-1/(RBD-VBD)
  Gain1 : Gain  Gain=-1
  Gain3 : Gain  Gain=-1
  Gravity : Gain  Gain=9.81
  Product : Product
  Rate Limiter : RateLimiter  RisingSlewLimit=1/tf  FallingSlewLimit=-1/tl  SampleTimeMode=inherited
  Relational Operator : RelationalOperator  OutDataTypeStr=boolean  RndMeth=Simplest
  Saturation : Saturate  UpperLimit=1  LowerLimit=0
  Saturation Dynamic : simulink/Discontinuities/Saturation Dynamic  OutMin=[]  OutMax=[]  OutDataTypeStr=Inherit: Same as second input  OutDataType=fixdt(1, 16)  OutScaling=2^-10  DoSatur=off
  Strahl formula : Polyval  Coefs=Pres
  Sum1 : Sum  Inputs=|+-
  Switch{,1..4} (5 alike) : Switch  Criteria=u2 ~= 0
  Transfer Fcn : TransferFcn  Numerator=BPnum  Denominator=BPden
  Transport Delay : TransportDelay  DelayTime=l/c  InitialOutput=p0
  efficiency : Product  Inputs=**
  friction coefficient : Constant  Value=fc
  lookup wagon braking efficiency : LookupNDDirect  TableIsInput=on
  lookup wagon mass : LookupNDDirect  TableIsInput=on
  max. braking force before slip : Product  Inputs=**
  "random index, generate once " : commrandsrc3/Random Integer Generator  SetSize=500  SeedSource=Auto  Seed=0  SampleTime=999999  SamplesPerFrame=1  OutputDataType=uint32  SimulateUsing=Interpreted execution
  track gradient : Bias  Bias=9.81*sin(trackgradient)
  v = v0 + a * t : Integrator  InitialConditionSource=external  InitialCondition=v0
  Fres : Outport  VectorParamsAs1DForOutWhenUnconnected=off
  p_BP_out : Outport  Port=2  VectorParamsAs1DForOutWhenUnconnected=off
  ares : Outport  Port=3
  m : Outport  Port=4
  "id " : Outport  Port=5
  wires:
  Strahl formula/1 -> Gravity/1
  Abs/1 -> Strahl formula/1
  Gravity/1 -> Product/2
  Product/1 -> Sum1/2  "Fw"
  v = v0 + a * t/1 -> Abs/1  "v"
  lookup wagon mass/1 -> Gain1/1, Switch3/1, max. braking force before slip/2, Divide/2, Product/1
  Divide/1 -> track gradient/1  "a"
  Gain/1 -> Saturation/1
  Fb/1 -> efficiency/2
  Saturation/1 -> Rate Limiter/1
  Rate Limiter/1 -> Fb/1
  Transfer Fcn/1 -> Dead Zone/1
  Transport Delay/1 -> Transfer Fcn/1
  efficiency/1 -> Sum1/1
  track gradient/1 -> Switch2/1, v = v0 + a * t/1  "ares"
  p/1 -> Gain/1, Transport Delay/1
  friction coefficient/1 -> max. braking force before slip/1
  Sum1/1 -> Saturation Dynamic/2  "Fres"
  Saturation Dynamic/1 -> Switch1/1, Divide/1
  max. braking force before slip/1 -> Saturation Dynamic/1, Gain3/1
  Gain3/1 -> Saturation Dynamic/3
  Data Store Read/1 -> v = v0 + a * t/2
  Dead Zone/1 -> Switch4/1
  Constant/1 -> lookup wagon braking efficiency/3, lookup wagon mass/3
  "random index, generate once "/1 -> Switch/1, lookup wagon mass/1, lookup wagon braking efficiency/1
  Constant1/1 -> lookup wagon mass/2
  Constant2/1 -> lookup wagon braking efficiency/2
  lookup wagon braking efficiency/1 -> efficiency/1
  Gain1/1 -> Fb/2
  Constant3/1 -> Relational Operator/1
  Constant4/1 -> Relational Operator/2
  Relational Operator/1 -> Switch1/2, Switch4/2, Switch2/2, Switch3/2, Switch/2
  Switch/1 -> "id "/1
  Constant5/1 -> Switch4/3, Switch1/3, Switch/3, Switch2/3, Switch3/3
  Switch1/1 -> Fres/1
  Switch2/1 -> ares/1
  Switch3/1 -> m/1
  Switch4/1 -> p_BP_out/1

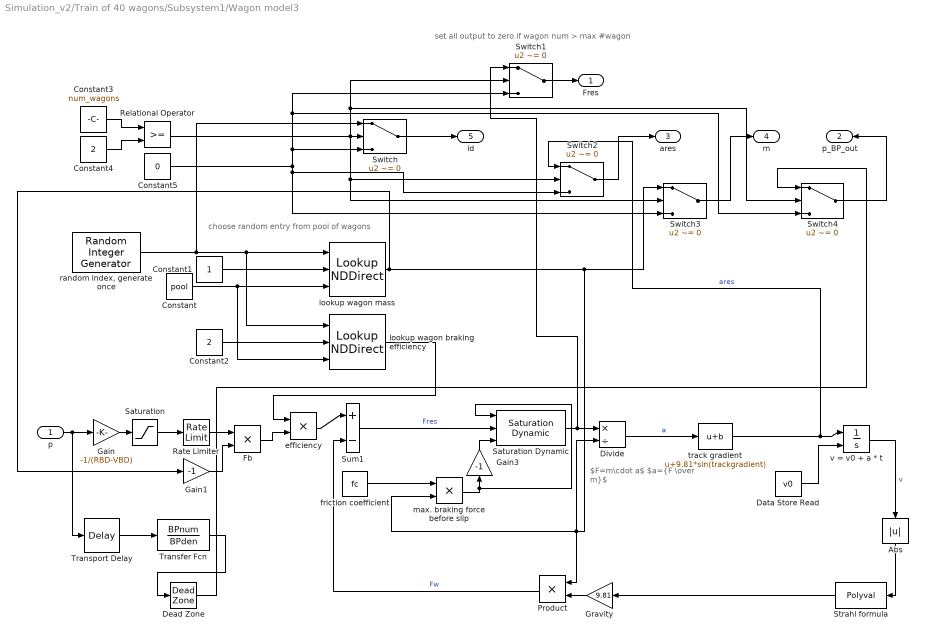
== system Simulation_v2/Train of 40 wagons/Subsystem1/Wagon model3 ==
  note: set all output to zero if wagon num > max #wagon
  note: choose random entry from pool of wagons
  note: $F=m\cdot a$ $a={F \over m}$
  p : Inport
  Abs : Abs
  Constant : Constant  Value=pool
  Constant1 : Constant
  Constant2 : Constant  Value=2
  Constant3 : Constant  Value=num_wagons
  Constant4 : Constant  Value=2
  Constant5 : Constant  Value=0  OutDataTypeStr=uint32
  Data Store Read : DataStoreRead  DataStoreName=v0
  Dead Zone : DeadZone  LowerValue=-0.005  UpperValue=0.005  SaturateOnIntegerOverflow=on
  Divide : Product  Inputs=*/
  Fb : Product  Inputs=**
  Gain : Gain  Gain=-1/(RBD-VBD)
  Gain1 : Gain  Gain=-1
  Gain3 : Gain  Gain=-1
  Gravity : Gain  Gain=9.81
  Product : Product
  Rate Limiter : RateLimiter  RisingSlewLimit=1/tf  FallingSlewLimit=-1/tl  SampleTimeMode=inherited
  Relational Operator : RelationalOperator  OutDataTypeStr=boolean  RndMeth=Simplest
  Saturation : Saturate  UpperLimit=1  LowerLimit=0
  Saturation Dynamic : simulink/Discontinuities/Saturation Dynamic  OutMin=[]  OutMax=[]  OutDataTypeStr=Inherit: Same as second input  OutDataType=fixdt(1, 16)  OutScaling=2^-10  DoSatur=off
  Strahl formula : Polyval  Coefs=Pres
  Sum1 : Sum  Inputs=|+-
  Switch{,1..4} (5 alike) : Switch  Criteria=u2 ~= 0
  Transfer Fcn : TransferFcn  Numerator=BPnum  Denominator=BPden
  Transport Delay : TransportDelay  DelayTime=l/c  InitialOutput=p0
  efficiency : Product  Inputs=**
  friction coefficient : Constant  Value=fc
  lookup wagon braking efficiency : LookupNDDirect  TableIsInput=on
  lookup wagon mass : LookupNDDirect  TableIsInput=on
  max. braking force before slip : Product  Inputs=**
  "random index, generate once " : commrandsrc3/Random Integer Generator  SetSize=500  SeedSource=Auto  Seed=0  SampleTime=999999  SamplesPerFrame=1  OutputDataType=uint32  SimulateUsing=Interpreted execution
  track gradient : Bias  Bias=9.81*sin(trackgradient)
  v = v0 + a * t : Integrator  InitialConditionSource=external  InitialCondition=v0
  Fres : Outport  VectorParamsAs1DForOutWhenUnconnected=off
  p_BP_out : Outport  Port=2  VectorParamsAs1DForOutWhenUnconnected=off
  ares : Outport  Port=3
  m : Outport  Port=4
  "id " : Outport  Port=5
  wires:
  Strahl formula/1 -> Gravity/1
  Abs/1 -> Strahl formula/1
  Gravity/1 -> Product/2
  Product/1 -> Sum1/2  "Fw"
  v = v0 + a * t/1 -> Abs/1  "v"
  lookup wagon mass/1 -> Gain1/1, Switch3/1, max. braking force before slip/2, Divide/2, Product/1
  Divide/1 -> track gradient/1  "a"
  Gain/1 -> Saturation/1
  Fb/1 -> efficiency/2
  Saturation/1 -> Rate Limiter/1
  Rate Limiter/1 -> Fb/1
  Transfer Fcn/1 -> Dead Zone/1
  Transport Delay/1 -> Transfer Fcn/1
  efficiency/1 -> Sum1/1
  track gradient/1 -> Switch2/1, v = v0 + a * t/1  "ares"
  p/1 -> Gain/1, Transport Delay/1
  friction coefficient/1 -> max. braking force before slip/1
  Sum1/1 -> Saturation Dynamic/2  "Fres"
  Saturation Dynamic/1 -> Switch1/1, Divide/1
  max. braking force before slip/1 -> Saturation Dynamic/1, Gain3/1
  Gain3/1 -> Saturation Dynamic/3
  Data Store Read/1 -> v = v0 + a * t/2
  Dead Zone/1 -> Switch4/1
  Constant/1 -> lookup wagon braking efficiency/3, lookup wagon mass/3
  "random index, generate once "/1 -> Switch/1, lookup wagon mass/1, lookup wagon braking efficiency/1
  Constant1/1 -> lookup wagon mass/2
  Constant2/1 -> lookup wagon braking efficiency/2
  lookup wagon braking efficiency/1 -> efficiency/1
  Gain1/1 -> Fb/2
  Constant3/1 -> Relational Operator/1
  Constant4/1 -> Relational Operator/2
  Relational Operator/1 -> Switch1/2, Switch4/2, Switch2/2, Switch3/2, Switch/2
  Switch/1 -> "id "/1
  Constant5/1 -> Switch4/3, Switch1/3, Switch/3, Switch2/3, Switch3/3
  Switch1/1 -> Fres/1
  Switch2/1 -> ares/1
  Switch3/1 -> m/1
  Switch4/1 -> p_BP_out/1

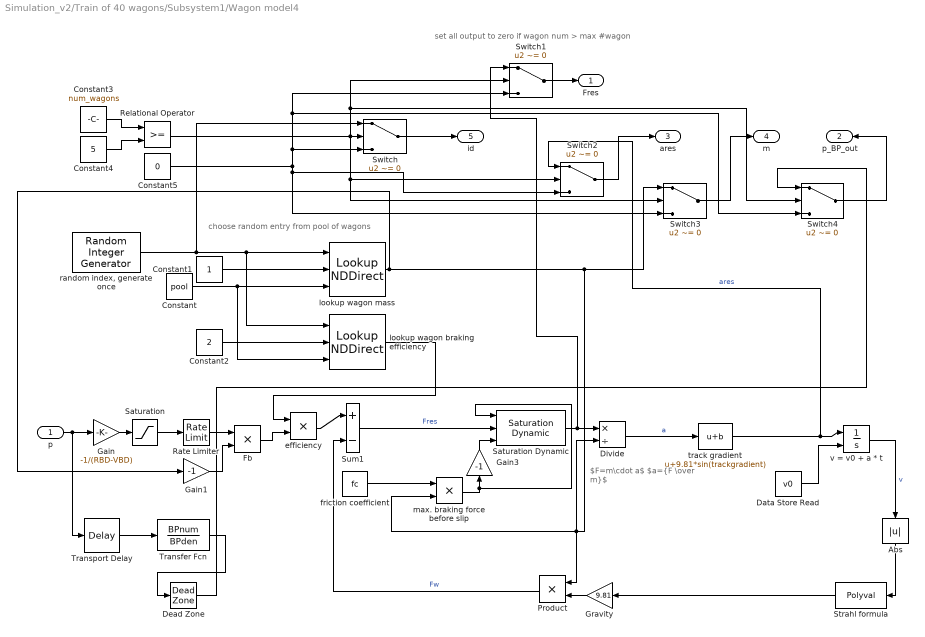
== system Simulation_v2/Train of 40 wagons/Subsystem1/Wagon model4 ==
  note: set all output to zero if wagon num > max #wagon
  note: choose random entry from pool of wagons
  note: $F=m\cdot a$ $a={F \over m}$
  p : Inport
  Abs : Abs
  Constant : Constant  Value=pool
  Constant1 : Constant
  Constant2 : Constant  Value=2
  Constant3 : Constant  Value=num_wagons
  Constant4 : Constant  Value=5
  Constant5 : Constant  Value=0  OutDataTypeStr=uint32
  Data Store Read : DataStoreRead  DataStoreName=v0
  Dead Zone : DeadZone  LowerValue=-0.005  UpperValue=0.005  SaturateOnIntegerOverflow=on
  Divide : Product  Inputs=*/
  Fb : Product  Inputs=**
  Gain : Gain  Gain=-1/(RBD-VBD)
  Gain1 : Gain  Gain=-1
  Gain3 : Gain  Gain=-1
  Gravity : Gain  Gain=9.81
  Product : Product
  Rate Limiter : RateLimiter  RisingSlewLimit=1/tf  FallingSlewLimit=-1/tl  SampleTimeMode=inherited
  Relational Operator : RelationalOperator  OutDataTypeStr=boolean  RndMeth=Simplest
  Saturation : Saturate  UpperLimit=1  LowerLimit=0
  Saturation Dynamic : simulink/Discontinuities/Saturation Dynamic  OutMin=[]  OutMax=[]  OutDataTypeStr=Inherit: Same as second input  OutDataType=fixdt(1, 16)  OutScaling=2^-10  DoSatur=off
  Strahl formula : Polyval  Coefs=Pres
  Sum1 : Sum  Inputs=|+-
  Switch{,1..4} (5 alike) : Switch  Criteria=u2 ~= 0
  Transfer Fcn : TransferFcn  Numerator=BPnum  Denominator=BPden
  Transport Delay : TransportDelay  DelayTime=l/c  InitialOutput=p0
  efficiency : Product  Inputs=**
  friction coefficient : Constant  Value=fc
  lookup wagon braking efficiency : LookupNDDirect  TableIsInput=on
  lookup wagon mass : LookupNDDirect  TableIsInput=on
  max. braking force before slip : Product  Inputs=**
  "random index, generate once " : commrandsrc3/Random Integer Generator  SetSize=500  SeedSource=Auto  Seed=0  SampleTime=999999  SamplesPerFrame=1  OutputDataType=uint32  SimulateUsing=Interpreted execution
  track gradient : Bias  Bias=9.81*sin(trackgradient)
  v = v0 + a * t : Integrator  InitialConditionSource=external  InitialCondition=v0
  Fres : Outport  VectorParamsAs1DForOutWhenUnconnected=off
  p_BP_out : Outport  Port=2  VectorParamsAs1DForOutWhenUnconnected=off
  ares : Outport  Port=3
  m : Outport  Port=4
  "id " : Outport  Port=5
  wires:
  Strahl formula/1 -> Gravity/1
  Abs/1 -> Strahl formula/1
  Gravity/1 -> Product/2
  Product/1 -> Sum1/2  "Fw"
  v = v0 + a * t/1 -> Abs/1  "v"
  lookup wagon mass/1 -> Gain1/1, Switch3/1, max. braking force before slip/2, Divide/2, Product/1
  Divide/1 -> track gradient/1  "a"
  Gain/1 -> Saturation/1
  Fb/1 -> efficiency/2
  Saturation/1 -> Rate Limiter/1
  Rate Limiter/1 -> Fb/1
  Transfer Fcn/1 -> Dead Zone/1
  Transport Delay/1 -> Transfer Fcn/1
  efficiency/1 -> Sum1/1
  track gradient/1 -> Switch2/1, v = v0 + a * t/1  "ares"
  p/1 -> Gain/1, Transport Delay/1
  friction coefficient/1 -> max. braking force before slip/1
  Sum1/1 -> Saturation Dynamic/2  "Fres"
  Saturation Dynamic/1 -> Switch1/1, Divide/1
  max. braking force before slip/1 -> Saturation Dynamic/1, Gain3/1
  Gain3/1 -> Saturation Dynamic/3
  Data Store Read/1 -> v = v0 + a * t/2
  Dead Zone/1 -> Switch4/1
  Constant/1 -> lookup wagon braking efficiency/3, lookup wagon mass/3
  "random index, generate once "/1 -> Switch/1, lookup wagon mass/1, lookup wagon braking efficiency/1
  Constant1/1 -> lookup wagon mass/2
  Constant2/1 -> lookup wagon braking efficiency/2
  lookup wagon braking efficiency/1 -> efficiency/1
  Gain1/1 -> Fb/2
  Constant3/1 -> Relational Operator/1
  Constant4/1 -> Relational Operator/2
  Relational Operator/1 -> Switch1/2, Switch4/2, Switch2/2, Switch3/2, Switch/2
  Switch/1 -> "id "/1
  Constant5/1 -> Switch4/3, Switch1/3, Switch/3, Switch2/3, Switch3/3
  Switch1/1 -> Fres/1
  Switch2/1 -> ares/1
  Switch3/1 -> m/1
  Switch4/1 -> p_BP_out/1

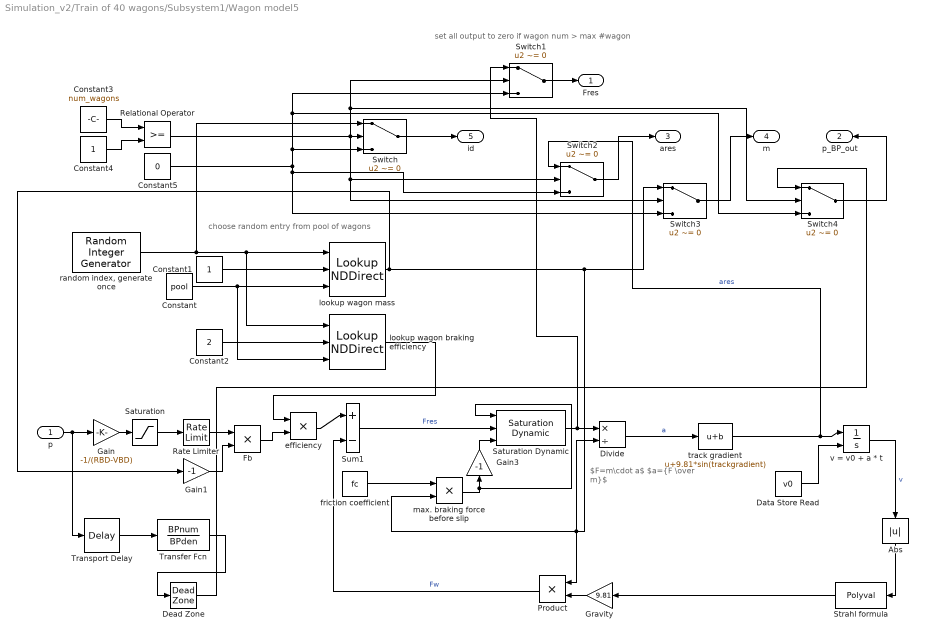
== system Simulation_v2/Train of 40 wagons/Subsystem1/Wagon model5 ==
  note: set all output to zero if wagon num > max #wagon
  note: choose random entry from pool of wagons
  note: $F=m\cdot a$ $a={F \over m}$
  p : Inport
  Abs : Abs
  Constant : Constant  Value=pool
  Constant1 : Constant
  Constant2 : Constant  Value=2
  Constant3 : Constant  Value=num_wagons
  Constant4 : Constant
  Constant5 : Constant  Value=0  OutDataTypeStr=uint32
  Data Store Read : DataStoreRead  DataStoreName=v0
  Dead Zone : DeadZone  LowerValue=-0.005  UpperValue=0.005  SaturateOnIntegerOverflow=on
  Divide : Product  Inputs=*/
  Fb : Product  Inputs=**
  Gain : Gain  Gain=-1/(RBD-VBD)
  Gain1 : Gain  Gain=-1
  Gain3 : Gain  Gain=-1
  Gravity : Gain  Gain=9.81
  Product : Product
  Rate Limiter : RateLimiter  RisingSlewLimit=1/tf  FallingSlewLimit=-1/tl  SampleTimeMode=inherited
  Relational Operator : RelationalOperator  OutDataTypeStr=boolean  RndMeth=Simplest
  Saturation : Saturate  UpperLimit=1  LowerLimit=0
  Saturation Dynamic : simulink/Discontinuities/Saturation Dynamic  OutMin=[]  OutMax=[]  OutDataTypeStr=Inherit: Same as second input  OutDataType=fixdt(1, 16)  OutScaling=2^-10  DoSatur=off
  Strahl formula : Polyval  Coefs=Pres
  Sum1 : Sum  Inputs=|+-
  Switch{,1..4} (5 alike) : Switch  Criteria=u2 ~= 0
  Transfer Fcn : TransferFcn  Numerator=BPnum  Denominator=BPden
  Transport Delay : TransportDelay  DelayTime=l/c  InitialOutput=p0
  efficiency : Product  Inputs=**
  friction coefficient : Constant  Value=fc
  lookup wagon braking efficiency : LookupNDDirect  TableIsInput=on
  lookup wagon mass : LookupNDDirect  TableIsInput=on
  max. braking force before slip : Product  Inputs=**
  "random index, generate once " : commrandsrc3/Random Integer Generator  SetSize=500  SeedSource=Auto  Seed=0  SampleTime=999999  SamplesPerFrame=1  OutputDataType=uint32  SimulateUsing=Interpreted execution
  track gradient : Bias  Bias=9.81*sin(trackgradient)
  v = v0 + a * t : Integrator  InitialConditionSource=external  InitialCondition=v0
  Fres : Outport  VectorParamsAs1DForOutWhenUnconnected=off
  p_BP_out : Outport  Port=2  VectorParamsAs1DForOutWhenUnconnected=off
  ares : Outport  Port=3
  m : Outport  Port=4
  "id " : Outport  Port=5
  wires:
  Strahl formula/1 -> Gravity/1
  Abs/1 -> Strahl formula/1
  Gravity/1 -> Product/2
  Product/1 -> Sum1/2  "Fw"
  v = v0 + a * t/1 -> Abs/1  "v"
  lookup wagon mass/1 -> Gain1/1, Switch3/1, max. braking force before slip/2, Divide/2, Product/1
  Divide/1 -> track gradient/1  "a"
  Gain/1 -> Saturation/1
  Fb/1 -> efficiency/2
  Saturation/1 -> Rate Limiter/1
  Rate Limiter/1 -> Fb/1
  Transfer Fcn/1 -> Dead Zone/1
  Transport Delay/1 -> Transfer Fcn/1
  efficiency/1 -> Sum1/1
  track gradient/1 -> Switch2/1, v = v0 + a * t/1  "ares"
  p/1 -> Gain/1, Transport Delay/1
  friction coefficient/1 -> max. braking force before slip/1
  Sum1/1 -> Saturation Dynamic/2  "Fres"
  Saturation Dynamic/1 -> Switch1/1, Divide/1
  max. braking force before slip/1 -> Saturation Dynamic/1, Gain3/1
  Gain3/1 -> Saturation Dynamic/3
  Data Store Read/1 -> v = v0 + a * t/2
  Dead Zone/1 -> Switch4/1
  Constant/1 -> lookup wagon braking efficiency/3, lookup wagon mass/3
  "random index, generate once "/1 -> Switch/1, lookup wagon mass/1, lookup wagon braking efficiency/1
  Constant1/1 -> lookup wagon mass/2
  Constant2/1 -> lookup wagon braking efficiency/2
  lookup wagon braking efficiency/1 -> efficiency/1
  Gain1/1 -> Fb/2
  Constant3/1 -> Relational Operator/1
  Constant4/1 -> Relational Operator/2
  Relational Operator/1 -> Switch1/2, Switch4/2, Switch2/2, Switch3/2, Switch/2
  Switch/1 -> "id "/1
  Constant5/1 -> Switch4/3, Switch1/3, Switch/3, Switch2/3, Switch3/3
  Switch1/1 -> Fres/1
  Switch2/1 -> ares/1
  Switch3/1 -> m/1
  Switch4/1 -> p_BP_out/1

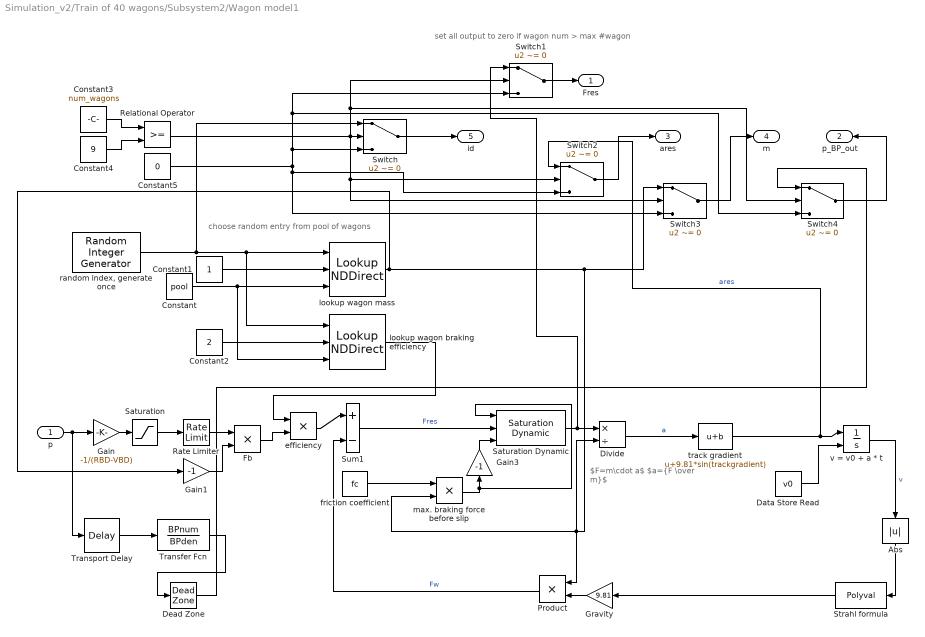
== system Simulation_v2/Train of 40 wagons/Subsystem2/Wagon model1 ==
  note: set all output to zero if wagon num > max #wagon
  note: choose random entry from pool of wagons
  note: $F=m\cdot a$ $a={F \over m}$
  p : Inport
  Abs : Abs
  Constant : Constant  Value=pool
  Constant1 : Constant
  Constant2 : Constant  Value=2
  Constant3 : Constant  Value=num_wagons
  Constant4 : Constant  Value=9
  Constant5 : Constant  Value=0  OutDataTypeStr=uint32
  Data Store Read : DataStoreRead  DataStoreName=v0
  Dead Zone : DeadZone  LowerValue=-0.005  UpperValue=0.005  SaturateOnIntegerOverflow=on
  Divide : Product  Inputs=*/
  Fb : Product  Inputs=**
  Gain : Gain  Gain=-1/(RBD-VBD)
  Gain1 : Gain  Gain=-1
  Gain3 : Gain  Gain=-1
  Gravity : Gain  Gain=9.81
  Product : Product
  Rate Limiter : RateLimiter  RisingSlewLimit=1/tf  FallingSlewLimit=-1/tl  SampleTimeMode=inherited
  Relational Operator : RelationalOperator  OutDataTypeStr=boolean  RndMeth=Simplest
  Saturation : Saturate  UpperLimit=1  LowerLimit=0
  Saturation Dynamic : simulink/Discontinuities/Saturation Dynamic  OutMin=[]  OutMax=[]  OutDataTypeStr=Inherit: Same as second input  OutDataType=fixdt(1, 16)  OutScaling=2^-10  DoSatur=off
  Strahl formula : Polyval  Coefs=Pres
  Sum1 : Sum  Inputs=|+-
  Switch{,1..4} (5 alike) : Switch  Criteria=u2 ~= 0
  Transfer Fcn : TransferFcn  Numerator=BPnum  Denominator=BPden
  Transport Delay : TransportDelay  DelayTime=l/c  InitialOutput=p0
  efficiency : Product  Inputs=**
  friction coefficient : Constant  Value=fc
  lookup wagon braking efficiency : LookupNDDirect  TableIsInput=on
  lookup wagon mass : LookupNDDirect  TableIsInput=on
  max. braking force before slip : Product  Inputs=**
  "random index, generate once " : commrandsrc3/Random Integer Generator  SetSize=500  SeedSource=Auto  Seed=0  SampleTime=999999  SamplesPerFrame=1  OutputDataType=uint32  SimulateUsing=Interpreted execution
  track gradient : Bias  Bias=9.81*sin(trackgradient)
  v = v0 + a * t : Integrator  InitialConditionSource=external  InitialCondition=v0
  Fres : Outport  VectorParamsAs1DForOutWhenUnconnected=off
  p_BP_out : Outport  Port=2  VectorParamsAs1DForOutWhenUnconnected=off
  ares : Outport  Port=3
  m : Outport  Port=4
  "id " : Outport  Port=5
  wires:
  Strahl formula/1 -> Gravity/1
  Abs/1 -> Strahl formula/1
  Gravity/1 -> Product/2
  Product/1 -> Sum1/2  "Fw"
  v = v0 + a * t/1 -> Abs/1  "v"
  lookup wagon mass/1 -> Gain1/1, Switch3/1, max. braking force before slip/2, Divide/2, Product/1
  Divide/1 -> track gradient/1  "a"
  Gain/1 -> Saturation/1
  Fb/1 -> efficiency/2
  Saturation/1 -> Rate Limiter/1
  Rate Limiter/1 -> Fb/1
  Transfer Fcn/1 -> Dead Zone/1
  Transport Delay/1 -> Transfer Fcn/1
  efficiency/1 -> Sum1/1
  track gradient/1 -> Switch2/1, v = v0 + a * t/1  "ares"
  p/1 -> Gain/1, Transport Delay/1
  friction coefficient/1 -> max. braking force before slip/1
  Sum1/1 -> Saturation Dynamic/2  "Fres"
  Saturation Dynamic/1 -> Switch1/1, Divide/1
  max. braking force before slip/1 -> Saturation Dynamic/1, Gain3/1
  Gain3/1 -> Saturation Dynamic/3
  Data Store Read/1 -> v = v0 + a * t/2
  Dead Zone/1 -> Switch4/1
  Constant/1 -> lookup wagon braking efficiency/3, lookup wagon mass/3
  "random index, generate once "/1 -> Switch/1, lookup wagon mass/1, lookup wagon braking efficiency/1
  Constant1/1 -> lookup wagon mass/2
  Constant2/1 -> lookup wagon braking efficiency/2
  lookup wagon braking efficiency/1 -> efficiency/1
  Gain1/1 -> Fb/2
  Constant3/1 -> Relational Operator/1
  Constant4/1 -> Relational Operator/2
  Relational Operator/1 -> Switch1/2, Switch4/2, Switch2/2, Switch3/2, Switch/2
  Switch/1 -> "id "/1
  Constant5/1 -> Switch4/3, Switch1/3, Switch/3, Switch2/3, Switch3/3
  Switch1/1 -> Fres/1
  Switch2/1 -> ares/1
  Switch3/1 -> m/1
  Switch4/1 -> p_BP_out/1
